simulink model "model_lab_3_on_off_control"  (R2021b)
settings: Solver=VariableStepAuto  StartTime=0.0  StopTime=4.5  RelTol=1e-3
model workspace (MAT data in the model file):
  U = 0
values from neighbouring files (symbols this model uses):
  DRAG = 0    [lab3_on_off.m]
  J = 0.0024    [lab3_on_off.m]
  Ke = 0.4870    (= 0.487)    [lab3_on_off.m]
  Km = 0.4870    (= 0.487)    [lab3_on_off.m]
  L = 0.0047    [lab3_on_off.m]
  R = 8.8696    [lab3_on_off.m]
  TARGET_ANGLE = 580    [lab3_on_off.m]
  VOLTAGE = 8.05    [lab3_on_off.m]
settings Model: Creator=huynh  LastModifiedBy=huynh

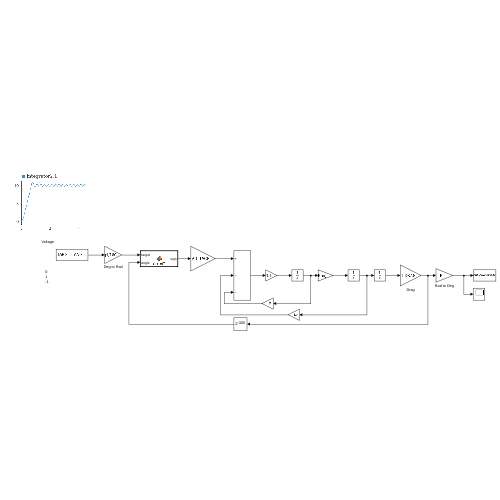
[thumbnail: Simulink's stored preview of the top-level diagram]
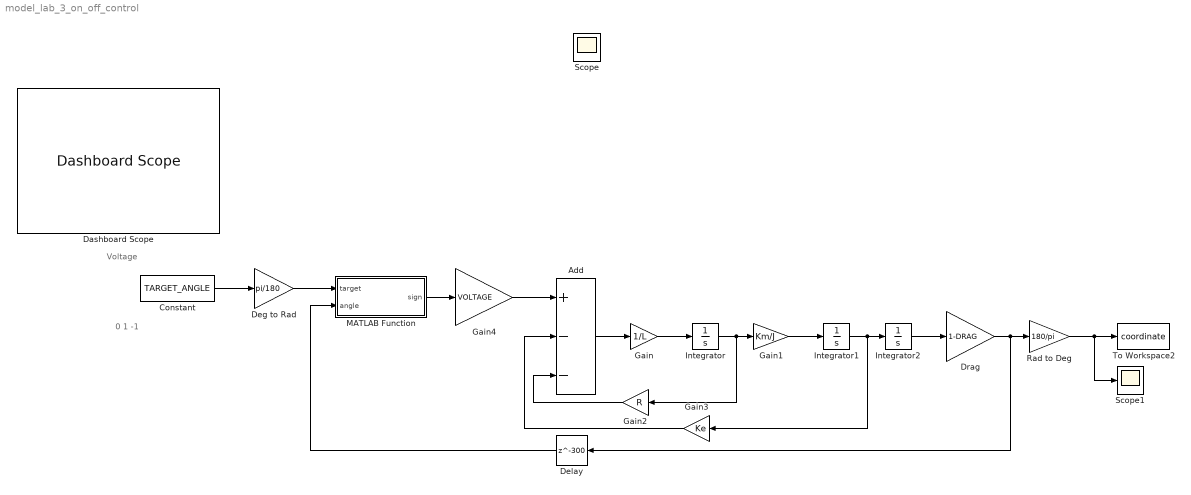
== system model_lab_3_on_off_control ==
  note: 0
      | 1
      | -1
  note: Voltage
  Add : Sum  Inputs=+--
  Constant : Constant  Value=TARGET_ANGLE
  Dashboard Scope : DashboardScope
  Deg to Rad : Gain  Gain=pi/180
  Delay : Delay  DelayLength=300  SampleTime=50e-6
  Drag : Gain  Gain=1-DRAG
  Gain : Gain  Gain=1/L
  Gain1 : Gain  Gain=Km/J
  Gain2 : Gain  Gain=R
  Gain3 : Gain  Gain=Ke
  Gain4 : Gain  Gain=VOLTAGE
  Integrator : Integrator
  Integrator1 : Integrator
  Integrator2 : Integrator
  MATLAB Function : MATLAB Function  TreatAsAtomicUnit=on
  Rad to Deg : Gain  Gain=180/pi
  Scope1 : Scope
  To Workspace2 : ToWorkspace  VariableName=coordinate  SaveFormat=Timeseries  SampleTime=-1
  Scope : Scope
  wires:
  Integrator1/1 -> Integrator2/1, Gain3/1
  Integrator/1 -> Gain2/1, Gain1/1
  Rad to Deg/1 -> To Workspace2/1, Scope1/1
  Gain/1 -> Integrator/1
  Gain1/1 -> Integrator1/1
  Gain2/1 -> Add/3
  Delay/1 -> MATLAB Function/2(angle)
  Integrator2/1 -> Drag/1
  Drag/1 -> Delay/1, Rad to Deg/1
  Gain4/1 -> Add/1
  Gain3/1 -> Add/2
  Deg to Rad/1 -> MATLAB Function/1(target)
  Add/1 -> Gain/1
  Constant/1 -> Deg to Rad/1
  MATLAB Function/1(sign) -> Gain4/1

== matlab function model_lab_3_on_off_control/MATLAB Function ==
  data: target input; angle input; sign output
function sign   = on_off(target, angle)
    sign = 0;
    if (angle < target) 
        sign = 1;
    end
    if (angle > target) 
        sign = -1; 
    end
    if (angle == target) 
        sign = 0;
    end
